simulink model "ex5"  (R2013a)
settings: Solver=ode45  StartTime=0.0  StopTime=10.0  RelTol=1e-3
values from neighbouring files (symbols this model uses):
  A = [0 0 1 0; 0 0 0 1; 0 566 -37 0; 0 -922 37 0]    [CEELab.m]    (also in ex1.m; ex11a.m; ex11b.m; ex2.m)
  b = [0 0 65 -65]'    [CEELab.m]    (also in ex1.m; ex11a.m; ex11b.m; ex3.m)
  c = [1 1 0 0]    [CEELab.m]    (also in ex11a.m; ex11b.m; ex2.m; ex3.m)
  K = (alphaK(2:5)-a(2:5))*inv(M)'*inv(CM)    [CEELab.m]    (also in ex11a.m; ex11b.m; ex4.m; labtotal.m = (alphac-a)*((M^-1)')*(C^-1))
  L = inv(OM)*inv(M)*(alphaL(2:5)-a(2:5))'    [CEELab.m]    (also in ex11a.m; ex11b.m; ex4.m; labtotal.m = (O^-1)*(M^-1)*(alphao-a)')
settings Model: Creator=João  LastModifiedBy=João

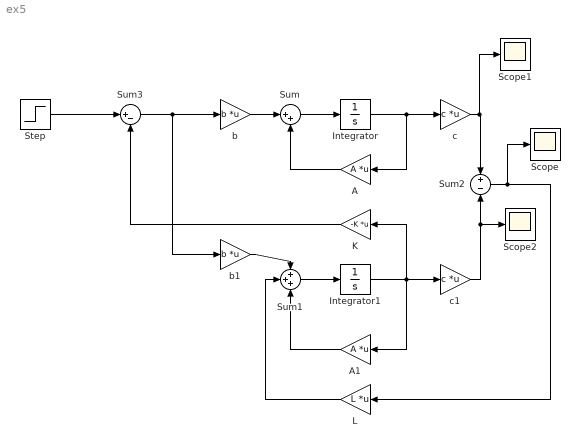
== system ex5 ==
  A : Gain  Gain=A  Multiplication=Matrix(K*u)
  A1 : Gain  Gain=A  Multiplication=Matrix(K*u)
  Integrator : Integrator
  Integrator1 : Integrator
  K : Gain  Gain=-K  Multiplication=Matrix(K*u)
  L : Gain  Gain=L  Multiplication=Matrix(K*u)
  Scope : Scope
  Scope1 : Scope
  Scope2 : Scope
      settings: SaveName=ScopeData2
  Step : Step  SampleTime=0
  Sum : Sum  Inputs=|++
  Sum1 : Sum  Inputs=+++
  Sum2 : Sum  Inputs=+-
  Sum3 : Sum  Inputs=|+-
  b : Gain  Gain=b  Multiplication=Matrix(K*u)
  b1 : Gain  Gain=b  Multiplication=Matrix(K*u)
  c : Gain  Gain=c  Multiplication=Matrix(K*u)
  c1 : Gain  Gain=c  Multiplication=Matrix(K*u)
  wires:
  Sum/1 -> Integrator/1
  b/1 -> Sum/1
  A/1 -> Sum/2
  Integrator/1 -> c/1, A/1
  Sum1/1 -> Integrator1/1
  Integrator1/1 -> K/1, c1/1, A1/1
  c1/1 -> Scope2/1, Sum2/2
  Sum2/1 -> Scope/1, L/1
  b1/1 -> Sum1/1
  L/1 -> Sum1/2
  A1/1 -> Sum1/3
  K/1 -> Sum3/2
  Sum3/1 -> b1/1, b/1
  c/1 -> Scope1/1, Sum2/1
  Step/1 -> Sum3/1
